simulink model "pathFollowingWithObstacleAvoidanceExample"  (R2020a)
settings: Solver=VariableStepAuto  StartTime=0.0  StopTime=inf  FixedStep=0.01  RelTol=1e-3  EnableMultiTasking=on
undefined symbols (not defined in the file or in its folder): Angular, Linear
libraries: robotlib x4, robotalgslib x2
settings Model: Creator=The MathWorks, Inc.  LastModifiedBy=Param
settings DataIOCC: ReturnWorkspaceOutputs=off
settings DebuggingCC: PregeneratedLibrarySubsystemCodeDiagnostic=none  ArithmeticOperatorsInVariantConditions=warning
settings SFSimCC: SimUseLocalCustomCode=off  CustomCodeUndefinedFunction=UseInterfaceOnly
settings RTWCC: RTWUseLocalCustomCode=off
settings CodeAppCC: StateflowObjectComments=on
settings GRTTargetCC: TargetLangStandard=C89/C90 (ANSI)
settings ConfigComp: CovMetricSettings=dsw  CovHtmlReporting=on  CovSaveCumulativeToWorkspaceVar=on  CovSaveSingleToWorkspaceVar=on  CovExternalEMLEnable=off

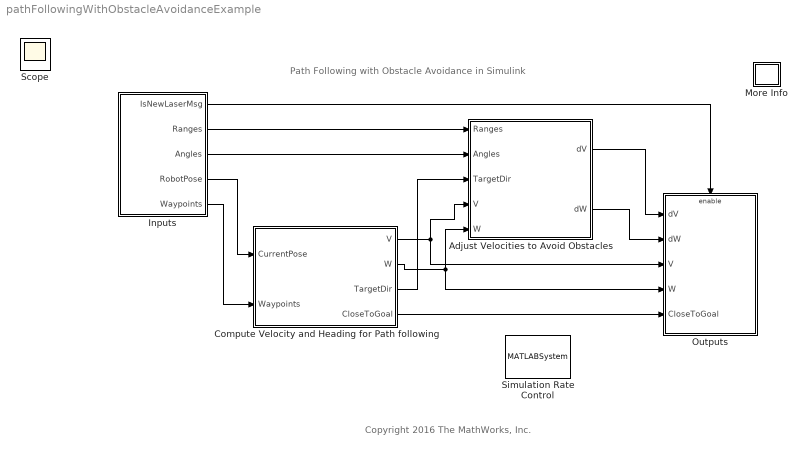
== system pathFollowingWithObstacleAvoidanceExample ==
  note: Path Following with Obstacle Avoidance in Simulink
  note: Copyright 2016 The MathWorks, Inc.
  Adjust Velocities to Avoid Obstacles : Subsystem
  Compute Velocity and Heading for Path following : Subsystem
  Inputs : Subsystem
  More Info : Subsystem
      settings: OpenFcn=showdemo(bdroot(gcb))
      mask Display: disp('?')
  Outputs : Subsystem
  Simulation Rate Control : MATLABSystem  System=ExampleHelperSimulationRateControl  SampleTime=0.02
      mask Type: ExampleHelperSimulationRateControl
      mask Display: disp('Rate Control');
  Scope : Scope
  wires:
  Compute Velocity and Heading for Path following/1(V) -> Outputs/3(V), Adjust Velocities to Avoid Obstacles/4(V)
  Compute Velocity and Heading for Path following/3(TargetDir) -> Adjust Velocities to Avoid Obstacles/3(TargetDir)
  Inputs/2(Ranges) -> Adjust Velocities to Avoid Obstacles/1(Ranges)
  Inputs/3(Angles) -> Adjust Velocities to Avoid Obstacles/2(Angles)
  Inputs/1(IsNewLaserMsg) -> Outputs/Enable
  Inputs/4(RobotPose) -> Compute Velocity and Heading for Path following/1(CurrentPose)
  Inputs/5(Waypoints) -> Compute Velocity and Heading for Path following/2(Waypoints)
  Compute Velocity and Heading for Path following/2(W) -> Outputs/4(W), Adjust Velocities to Avoid Obstacles/5(W)
  Adjust Velocities to Avoid Obstacles/1(dV) -> Outputs/1(dV)
  Adjust Velocities to Avoid Obstacles/2(dW) -> Outputs/2(dW)
  Compute Velocity and Heading for Path following/4(CloseToGoal) -> Outputs/5(CloseToGoal)

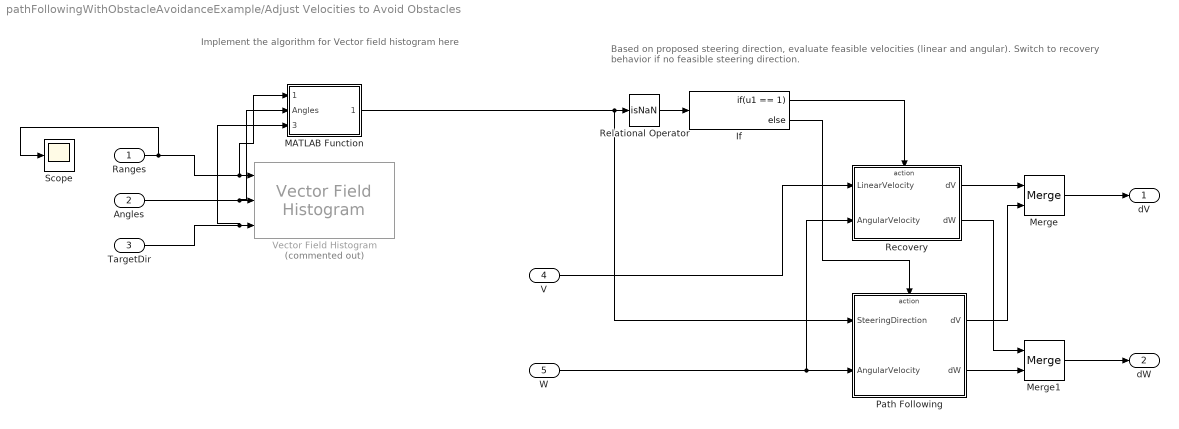
== system pathFollowingWithObstacleAvoidanceExample/Adjust Velocities to Avoid Obstacles ==
  note: Implement the algorithm for Vector field histogram here
  note: Based on proposed steering direction, evaluate feasible velocities (linear and angular).
      | 				Switch to recovery behavior if no feasible steering direction.
  Ranges : Inport
  Angles : Inport  Port=2
  TargetDir : Inport  Port=3
  V : Inport  Port=4
  W : Inport  Port=5
  If : If  IfExpression=u1 == 1
  MATLAB Function : MATLAB Function  TreatAsAtomicUnit=on
  Merge : Merge
  Merge1 : Merge
  Path Following : Subsystem  TreatAsAtomicUnit=on
  Recovery : Subsystem  TreatAsAtomicUnit=on
  Relational Operator : RelationalOperator  Operator=isNaN  OutDataTypeStr=boolean  RndMeth=Simplest
  Scope : Scope
  Vector Field Histogram : robotalgslib/Vector Field Histogram  Commented=on  NumAngularSectors=180  DistanceLimits=[ 0.05, 2 ]  HistogramThresholds=[ 3, 10 ]  RobotRadius=0.1  SafetyDistance=0.1  MinTurningRadius=0.1  SimulateUsing=Code generation  TargetDirectionWeight=5  CurrentDirectionWeight=2  PreviousDirectionWeight=2
      settings: SourceProductBaseCode=NV,RO
  dV : Outport  VectorParamsAs1DForOutWhenUnconnected=off
  dW : Outport  Port=2  VectorParamsAs1DForOutWhenUnconnected=off
  wires:
  Merge1/1 -> dW/1
  V/1 -> Recovery/1(LinearVelocity)
  W/1 -> Recovery/2(AngularVelocity), Path Following/2(AngularVelocity)
  Relational Operator/1 -> If/1
  Merge/1 -> dV/1
  If/1 -> Recovery/Action
  If/2 -> Path Following/Action
  Recovery/2(dW) -> Merge1/1
  Path Following/2(dW) -> Merge1/2
  Recovery/1(dV) -> Merge/1
  Path Following/1(dV) -> Merge/2
  Ranges/1 -> Scope/1, MATLAB Function/1(Ranges), Vector Field Histogram/1
  Angles/1 -> MATLAB Function/2(Angles), Vector Field Histogram/2
  TargetDir/1 -> MATLAB Function/3(TargetDir), Vector Field Histogram/3
  MATLAB Function/1(outangle) -> Path Following/1(SteeringDirection), Relational Operator/1

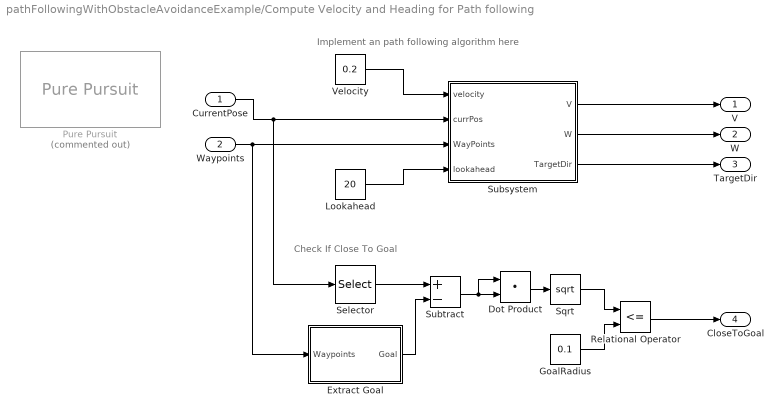
== system pathFollowingWithObstacleAvoidanceExample/Compute Velocity and Heading for Path following ==
  note: Implement an path following algorithm here
  note: Check If Close To Goal
  CurrentPose : Inport
  Waypoints : Inport  Port=2
  " Extract Goal" : MATLAB Function  TreatAsAtomicUnit=on
  Dot Product : DotProduct  InputSameDT=on  OutDataTypeStr=Inherit: Inherit via internal rule
  GoalRadius : Constant  Value=0.1
  Lookahead : Constant  Value=20  OutDataTypeStr=Inherit: Inherit via back propagation
  Pure Pursuit : robotalgslib/Pure Pursuit  Commented=on  DesiredLinearVelocity=0.1  MaxAngularVelocity=1.0  LookaheadDistance=1.0  TargetDirPort=on  SimulateUsing=Code generation
  Relational Operator : RelationalOperator  Operator=<=  OutDataTypeStr=boolean  RndMeth=Simplest
  Selector : Selector  InputPortWidth=3  IndexOptions=Index vector (dialog)  Indices=[1 2]  OutputSizes=1
  Sqrt : Sqrt  SaturateOnIntegerOverflow=on
  Subsystem : Subsystem
  Subtract : Sum  Inputs=+-
  Velocity : Constant  Value=0.2  OutDataTypeStr=Inherit: Inherit via back propagation
  V : Outport  VectorParamsAs1DForOutWhenUnconnected=off
  W : Outport  Port=2  VectorParamsAs1DForOutWhenUnconnected=off
  TargetDir : Outport  Port=3  VectorParamsAs1DForOutWhenUnconnected=off
  CloseToGoal : Outport  Port=4  VectorParamsAs1DForOutWhenUnconnected=off
  wires:
  " Extract Goal"/1(Goal) -> Subtract/2
  Waypoints/1 -> Subsystem/3(WayPoints), " Extract Goal"/1(Waypoints)
  CurrentPose/1 -> Subsystem/2(currPos), Selector/1
  Relational Operator/1 -> CloseToGoal/1
  GoalRadius/1 -> Relational Operator/2
  Selector/1 -> Subtract/1
  Dot Product/1 -> Sqrt/1
  Sqrt/1 -> Relational Operator/1
  Subtract/1 -> Dot Product/1, Dot Product/2
  Velocity/1 -> Subsystem/1(velocity)
  Lookahead/1 -> Subsystem/4(lookahead)
  Subsystem/3(TargetDir) -> TargetDir/1
  Subsystem/1(V) -> V/1
  Subsystem/2(W) -> W/1

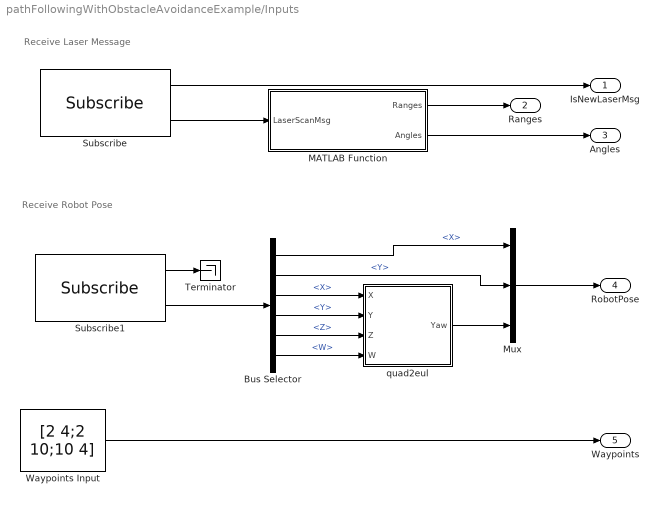
== system pathFollowingWithObstacleAvoidanceExample/Inputs ==
  note: Receive Robot Pose
  note: Receive Laser Message
  Bus Selector : BusSelector  OutputSignals=Pose.Pose.Position.X,Pose.Pose.Position.Y,Pose.Pose.Orientation.X,Pose.Pose.Orientation.Y,Pose.Pose.Orientation.Z,Pose.Pose.Orientation.W
  MATLAB Function : MATLAB Function  TreatAsAtomicUnit=on
  Mux : Mux  Inputs=3
  Subscribe : robotlib/Subscribe  topicSource=Select from ROS network  topic=/scan  messageType=sensor_msgs/LaserScan  sampleTime=-1  messageQueueLength=1
  Subscribe1 : robotlib/Subscribe  topicSource=Select from ROS network  topic=/ground_truth_pose  messageType=nav_msgs/Odometry  sampleTime=-1  messageQueueLength=1
  Terminator : Terminator
  Waypoints Input : Constant  Value=[2 4;2 10;10 4]  VectorParams1D=off  OutDataTypeStr=double
  quad2eul : MATLAB Function  TreatAsAtomicUnit=on
  IsNewLaserMsg : Outport  VectorParamsAs1DForOutWhenUnconnected=off
  Ranges : Outport  Port=2  VectorParamsAs1DForOutWhenUnconnected=off
  Angles : Outport  Port=3  VectorParamsAs1DForOutWhenUnconnected=off
  RobotPose : Outport  Port=4  VectorParamsAs1DForOutWhenUnconnected=off
  Waypoints : Outport  Port=5  VectorParamsAs1DForOutWhenUnconnected=off
  wires:
  Waypoints Input/1 -> Waypoints/1
  Subscribe/2 -> MATLAB Function/1(LaserScanMsg)
  quad2eul/1(Yaw) -> Mux/3
  Subscribe1/2 -> Bus Selector/1
  Bus Selector/3 -> quad2eul/1(X)  "<X>"
  Subscribe1/1 -> Terminator/1
  Bus Selector/2 -> Mux/2  "<Y>"
  Bus Selector/5 -> quad2eul/3(Z)  "<Z>"
  Bus Selector/4 -> quad2eul/2(Y)  "<Y>"
  Bus Selector/1 -> Mux/1  "<X>"
  Bus Selector/6 -> quad2eul/4(W)  "<W>"
  MATLAB Function/1(Ranges) -> Ranges/1
  MATLAB Function/2(Angles) -> Angles/1
  Subscribe/1 -> IsNewLaserMsg/1
  Mux/1 -> RobotPose/1

== system pathFollowingWithObstacleAvoidanceExample/More Info ==

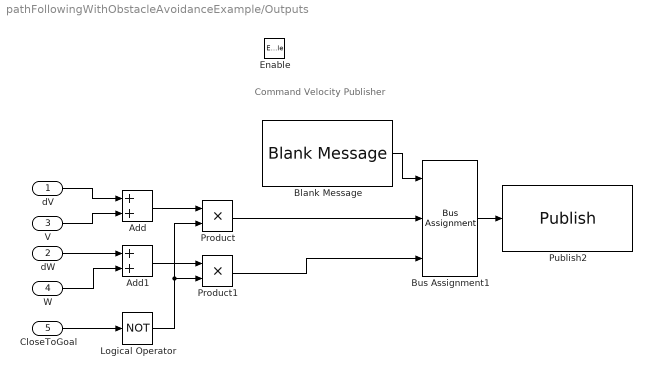
== system pathFollowingWithObstacleAvoidanceExample/Outputs ==
  note: Command Velocity Publisher
  dV : Inport
  dW : Inport  Port=2
  V : Inport  Port=3
  W : Inport  Port=4
  CloseToGoal : Inport  Port=5
  Enable : EnablePort
  Add : Sum
  Add1 : Sum
  Blank Message : robotlib/Blank Message  messageClass=Message  entityType=geometry_msgs/Twist  messageType=geometry_msgs/Twist  SampleTime=inf
  Bus Assignment1 : BusAssignment  DialogController=Simulink.DDGSource_BusAssignment  AssignedSignals=Linear.X,Angular.Z
  Logical Operator : Logic  Operator=NOT  AllPortsSameDT=off  OutDataTypeStr=boolean
  Product : Product
  Product1 : Product
  Publish2 : robotlib/Publish  topicSource=Select from ROS network  topic=/mobile_base/commands/velocity  messageType=geometry_msgs/Twist  messageQueueLength=105
  wires:
  V/1 -> Add/2
  W/1 -> Add1/2
  dV/1 -> Add/1
  dW/1 -> Add1/1
  CloseToGoal/1 -> Logical Operator/1
  Add/1 -> Product/1
  Add1/1 -> Product1/1
  Product1/1 -> Bus Assignment1/3
  Product/1 -> Bus Assignment1/2
  Blank Message/1 -> Bus Assignment1/1
  Bus Assignment1/1 -> Publish2/1
  Logical Operator/1 -> Product1/2, Product/2

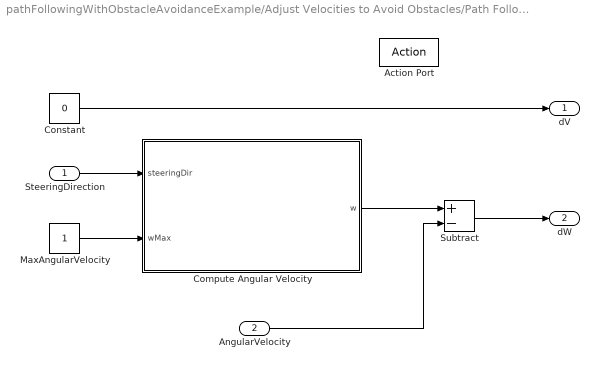
== system pathFollowingWithObstacleAvoidanceExample/Adjust Velocities to Avoid Obstacles/Path Following ==
  SteeringDirection : Inport
  AngularVelocity : Inport  Port=2
  Action Port : ActionPort  ActionPortLabel=else
  Compute Angular Velocity : MATLAB Function  TreatAsAtomicUnit=on
  Constant : Constant  Value=0
  MaxAngularVelocity : Constant
  Subtract : Sum  Inputs=+-
  dV : Outport  VectorParamsAs1DForOutWhenUnconnected=off
  dW : Outport  Port=2  VectorParamsAs1DForOutWhenUnconnected=off
  wires:
  Constant/1 -> dV/1
  MaxAngularVelocity/1 -> Compute Angular Velocity/2(wMax)
  SteeringDirection/1 -> Compute Angular Velocity/1(steeringDir)
  Subtract/1 -> dW/1
  Compute Angular Velocity/1(w) -> Subtract/1
  AngularVelocity/1 -> Subtract/2

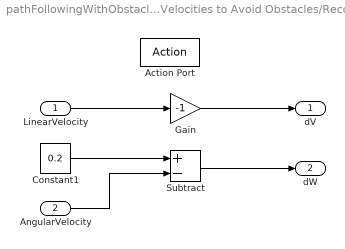
== system pathFollowingWithObstacleAvoidanceExample/Adjust Velocities to Avoid Obstacles/Recovery ==
  LinearVelocity : Inport
  AngularVelocity : Inport  Port=2
  Action Port : ActionPort  ActionPortLabel=if(u1 == 1)
  Constant1 : Constant  Value=0.2
  Gain : Gain  Gain=-1
  Subtract : Sum  Inputs=+-
  dV : Outport  VectorParamsAs1DForOutWhenUnconnected=off
  dW : Outport  Port=2  VectorParamsAs1DForOutWhenUnconnected=off
  wires:
  LinearVelocity/1 -> Gain/1
  Gain/1 -> dV/1
  Constant1/1 -> Subtract/1
  AngularVelocity/1 -> Subtract/2
  Subtract/1 -> dW/1

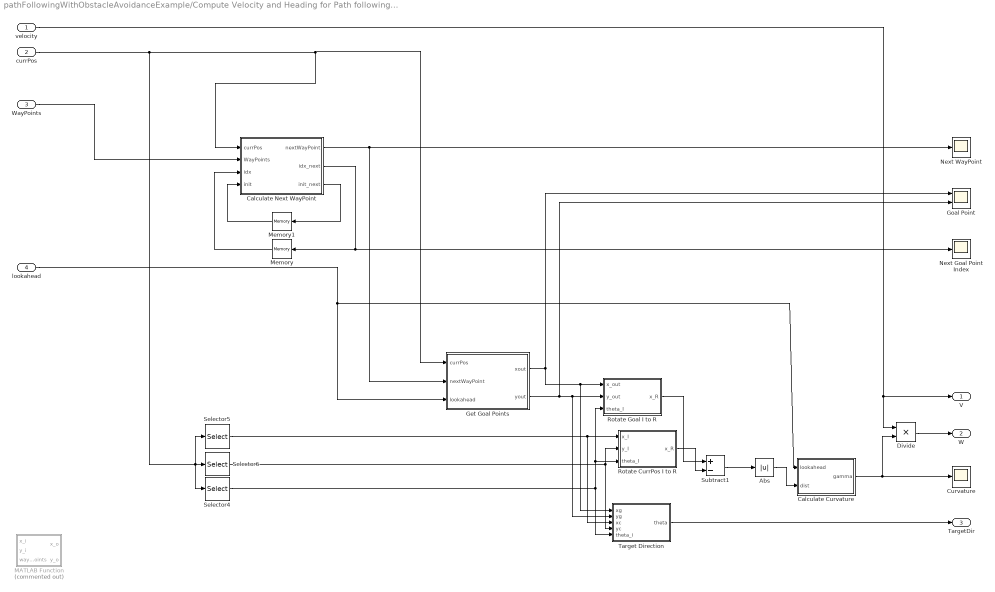
== system pathFollowingWithObstacleAvoidanceExample/Compute Velocity and Heading for Path following/Subsystem ==
  velocity : Inport
  currPos : Inport  Port=2
  WayPoints : Inport  Port=3
  lookahead : Inport  Port=4
  " Rotate CurrPos I to R" : MATLAB Function  TreatAsAtomicUnit=on
  " Rotate Goal I to R" : MATLAB Function  TreatAsAtomicUnit=on
  Abs : Abs
  Calculate Curvature : MATLAB Function  TreatAsAtomicUnit=on
  Calculate Next WayPoint : MATLAB Function  TreatAsAtomicUnit=on
  Curvature : Scope
  Divide : Product  Inputs=**
  Get Goal Points : MATLAB Function  TreatAsAtomicUnit=on
  Goal Point : Scope  NumInputPorts=2
  MATLAB Function : MATLAB Function  Commented=on  TreatAsAtomicUnit=on
  Memory : Memory  InitialCondition=1
  Memory1 : Memory
  Next Goal Point Index : Scope
  Next WayPoint : Scope
  Selector4 : Selector  InputPortWidth=3  IndexOptions=Index vector (dialog)  Indices=[3]  OutputSizes=1
  Selector5 : Selector  InputPortWidth=3  IndexOptions=Index vector (dialog)  Indices=[1]  OutputSizes=1
  Selector6 : Selector  InputPortWidth=3  IndexOptions=Index vector (dialog)  Indices=[2]  OutputSizes=1
  Subtract1 : Sum  Inputs=+-
  Target Direction : MATLAB Function  TreatAsAtomicUnit=on
  V : Outport  VectorParamsAs1DForOutWhenUnconnected=off
  W : Outport  Port=2  VectorParamsAs1DForOutWhenUnconnected=off
  TargetDir : Outport  Port=3  VectorParamsAs1DForOutWhenUnconnected=off
  wires:
  lookahead/1 -> Get Goal Points/3(lookahead), Calculate Curvature/1(lookahead)
  velocity/1 -> V/1, Divide/1
  Calculate Next WayPoint/1(nextWayPoint) -> Get Goal Points/2(nextWayPoint), Next WayPoint/1
  currPos/1 -> Get Goal Points/1(currPos), Calculate Next WayPoint/1(currPos), Selector4/1, Selector5/1, Selector6/1
  Selector5/1 -> " Rotate CurrPos I to R"/1(x_I), Target Direction/3(xc)
  WayPoints/1 -> Calculate Next WayPoint/2(WayPoints)
  Selector4/1 -> Target Direction/5(theta_i), " Rotate CurrPos I to R"/3(theta_I), " Rotate Goal I to R"/3(theta_I)
  Selector6/1 -> " Rotate CurrPos I to R"/2(y_I), Target Direction/4(yc)
  Abs/1 -> Calculate Curvature/2(dist)
  " Rotate Goal I to R"/1(x_R) -> Subtract1/1
  " Rotate CurrPos I to R"/1(x_R) -> Subtract1/2
  Calculate Curvature/1(gamma) -> Divide/2, Curvature/1
  Target Direction/1(theta) -> TargetDir/1
  Subtract1/1 -> Abs/1
  Divide/1 -> W/1
  Calculate Next WayPoint/2(idx_next) -> Next Goal Point Index/1, Memory/1
  Get Goal Points/1(xout) -> " Rotate Goal I to R"/1(x_out), Target Direction/1(xg), Goal Point/1
  Get Goal Points/2(yout) -> " Rotate Goal I to R"/2(y_out), Target Direction/2(yg), Goal Point/2
  Memory/1 -> Calculate Next WayPoint/3(idx)
  Calculate Next WayPoint/3(init_next) -> Memory1/1
  Memory1/1 -> Calculate Next WayPoint/4(init)

== matlab function pathFollowingWithObstacleAvoidanceExample/Compute Velocity and Heading for Path following/Subsystem/Target Direction ==
  data: xg input; yg input; theta output; xc input; yc input; theta_i input
function theta = targetDir(xg,yg,xc,yc,theta_i)
%#codegen
theta = angdiff(theta_i,atan2(yg-yc,xg-xc));
end

== matlab function pathFollowingWithObstacleAvoidanceExample/Adjust Velocities to Avoid Obstacles/MATLAB Function ==
  data: Ranges input; Angles input; TargetDir input; outangle output
function outangle = steeringAngle(Ranges,Angles,TargetDir)
disp("--")
badindices = bitor(isnan(Ranges),isnan(Angles));
Ranges = Ranges(~badindices);
Angles = Angles(~badindices);
a = 15;
b = 1;
Ranges = a-b*Ranges;
numBins = 60; 
edges = linspace(-pi/2,pi/2,numBins+1);
validindices = bitand(Angles >= -pi/2, Angles <= pi/2);
Ranges = Ranges(validindices);
Angles = Angles(validindices);
disp(edges)
[~,edges,bin]=histcounts(Angles,edges);
disp("bin value")
disp(bin)
B = accumarray(bin,Ranges,[numBins 1]);
B = conv(B,1/7*[1 2 3 2 1], 'same');
% B = conv(B,1/11*[1 2 3 4 5 4 3 2 1], 'same');
disp(size(bin))
disp(size(Ranges))
disp("B value")
disp(B)
[~,~,idx]=histcounts(TargetDir,edges);
idx = max(1,idx);
idx = min(idx,numBins);
% minbins with 0 values 
threshold = 15
Bnew = conv(B,1/7*[1 1 1 1 1 1 1], 'same');
disp("Bnew value")
disp(Bnew)
indices = find(Bnew<=threshold);
if isempty(indices)
    outangle = pi/18
else
    [minval, minidx] = min(abs(indices-idx));
        startx = 1;
        endx = size(indices,1);
        if indices(minidx)>=idx
            startx = indices(minidx);
            i = indices(minidx);
            while (Bnew(i)<=threshold & i<size(Bnew))
                endx = i;
                i = i+1;
            end
            outangle = (0.9*edges(startx)+0.1*edges(endx+1))/2;
        else
            endx = indices(minidx);
            i = indices(minidx);
            while (Bnew(i)<=threshold & i>1)
                startx = i;
                i = i-1;
            end
            outangle = (0.1*edges(startx)+0.9*edges(endx+1))/2;
        end
end
disp(idx)
disp(TargetDir)
disp(outangle)

== matlab function pathFollowingWithObstacleAvoidanceExample/Inputs/quad2eul ==
  data: X input; Yaw output; Y input; Z input; W input
function Yaw = quat2eulBlk(X, Y, Z, W)
%#codegen

eularAngles = quat2eul([W, X, Y, Z]);
Yaw = eularAngles(1);

== matlab function pathFollowingWithObstacleAvoidanceExample/Compute Velocity and Heading for Path following/Subsystem/MATLAB Function ==
  data: x_i input; x_o output; y_i input; waypoints input; y_o output
function [x_o, y_o] = pathpoint(x_i, y_i, waypoints)
    distances = pdist2([x_i, y_i],waypoints);
    [minDistance, indexOfMinDistance] = min(distances);
    idx = indexOfMinDistance;
    if indexOfMinDistance == size(waypoints,1)
        idx = idx - 1;
    end
    coefficients = polyfit(distances[indexOfMinDistance],distances[indexOfMinDistance+1], 1);
    m = coefficients(1);
    c = coefficients(2);
    refPath = referencePathFrenet(waypoints);

    
y = u;

== matlab function pathFollowingWithObstacleAvoidanceExample/Compute Velocity and Heading for Path following/Subsystem/ Rotate CurrPos I to R ==
  data: x_I input; y_I input; x_R output; theta_I input
function x_R  = rotation(x_I,y_I,theta_I)
%#codegen
x_R = x_I*cos(theta_I)+y_I*sin(theta_I);
% y_R = -x_I*sin(theta_I)+y_I*cos(theta_I);
% theta_R = theta_I;

== matlab function pathFollowingWithObstacleAvoidanceExample/Compute Velocity and Heading for Path following/Subsystem/Get Goal Points ==
  data: currPos input; xout output; nextWayPoint input; yout output; lookahead input
function [xout,yout] = getGoalPos(currPos,nextWayPoint,lookahead)
x1 = currPos(1);
y1 = currPos(2);
x2 = nextWayPoint(1);
y2 = nextWayPoint(2);
dist = pdist([x1,y1;x2,y2],'euclidean');

if dist<lookahead
    xout = x2;
    yout = y2;
else
    xout = x1+(lookahead/dist)*(x2-x1);
    yout = y1+(lookahead/dist)*(y2-y1);
end
disp("===")
disp([x1,y1;x2,y2;xout,yout])
% eps = 1e-8;
% slope = (y2-y1)/(x2-x1+eps);
% intercpt = (y1*x2-y2*x1)/(x2-x1+eps);

% [xout,yout] = linecirc(slope,intercpt,x1,x2,lookahead);
% fun1 = @(x)(x-x1)^2+(slope*x+intercpt-y1)^2-lookahead^2;
% if fun1(x1)*fun1(x2)>0
%     xout = x2;
%     yout = y2;
% else
%     xout = fzero(fun1,[x1,x2]);
%     yout = slope*xout+intercpt;
% end

== matlab function pathFollowingWithObstacleAvoidanceExample/Inputs/MATLAB Function ==
  data: LaserScanMsg input; Ranges output; Angles output
function [Ranges, Angles] = ExtractRangeData(LaserScanMsg)
%#codegen

% Extract Range information
Ranges = double(LaserScanMsg.Ranges);

% Construct Angles vector using AngleMin and AngleIncrement from sensor
% reading.
angMin = double(LaserScanMsg.AngleMin);
angIncrement = double(LaserScanMsg.AngleIncrement);

numReadings = numel(Ranges);
rawAngles = angMin + (0:numReadings-1)' * angIncrement;

% Wrap the angles to the (-pi,pi] interval.
Angles = robotics.internal.wrapToPi(double(rawAngles));

== matlab function pathFollowingWithObstacleAvoidanceExample/Compute Velocity and Heading for Path following/Subsystem/Calculate Next WayPoint ==
  data: currPos input; nextWayPoint output; WayPoints input; idx input; idx_next output; init input; init_next output
function [nextWayPoint, idx_next, init_next] = nextWayPoint(currPos,WayPoints,idx, init)
init_next = init
if init == 0
    distances = pdist2(currPos(1:2)',WayPoints(idx,:));
    [minDistance, minidx] = min(distances);
    idx = minidx
    init_next = 1
end
idx_next = idx
if norm(currPos(1:2)'-WayPoints(idx,:))<0.1
    idx_next = min(idx + 1, size(WayPoints, 1))
end
nextWayPoint = WayPoints(idx_next,:);
end

== matlab function pathFollowingWithObstacleAvoidanceExample/Compute Velocity and Heading for Path following/ Extract Goal ==
  data: Waypoints input; Goal output
function Goal = extractGoal(Waypoints)
%#codegen
b = isnan(Waypoints);
[rows,~] = find(b);
ridx = setdiff(1:size(Waypoints,1), sort(rows));
Goal = [Waypoints(ridx(end), 1) Waypoints(ridx(end), 2)];

== matlab function pathFollowingWithObstacleAvoidanceExample/Adjust Velocities to Avoid Obstacles/Path Following/Compute Angular Velocity ==
  data: steeringDir input; w output; wMax input
function w = exampleHelperComputeAngularVelocity(steeringDir, wMax)
%EXAMPLEHELPERCOMPUTEANGULARVELOCITY Compute angular velocity
%   W = exampleHelperComputeAngularVelocity(STEERINGDIR)
%   returns the angular velocity W for a differential drive robot in radians
%   per second for a given steering direction STEERINGDIR in the robot's
%   coordinate frame in radians.
%
%   W = exampleHelperComputeAngularVelocity(STEERINGDIR, WMAX)
%   returns the angular velocity W for a differential drive robot in radians
%   per second for a given steering direction STEERINGDIR in the robot's
%   coordinate frame in radians and maximum angular velocity WMAX in
%   radians per second. The output angular velocity is saturated based on
%   the WMAX.
%
%   Example:
%       
%       w = exampleHelperComputeAngularVelocity(0.2, 1);

% Copyright 2015 The MathWorks, Inc.

%#codegen
%#ok<*EMCA>

% Allow variable input arguments
if nargin == 1   
    wMax = inf;
end

validateattributes(steeringDir, {'double'},{'real'},...
    'exampleHelperComputeAngularVelocity', 'STEERINGDIR', 1);
validateattributes(wMax, {'double'},{'real', 'positive'},...
    'exampleHelperComputeAngularVelocity', 'WMAX', 2);

% Computing in robot's coordinate frame
curPose = [0 0 0];

% The following computation is similar to robotics.PurePursuit
lookaheadPoint = [cos(steeringDir), sin(steeringDir)];
slope = atan2((lookaheadPoint(2) - curPose(2)), ...
    (lookaheadPoint(1) - curPose(1)));
alpha = angdiff(curPose(3), slope);

% Angular velocity command for a differential drive robot is
% equal to the desired curvature to be followed by the robot.

w = (2*sin(alpha));

% Pick a constant rotation when robot is facing in the opposite
% direction of the path
if abs(abs(alpha) - pi) < 1e-12
    w = sign(w)*1;
end

if abs(w) > wMax
    w = sign(w)*wMax;
end

end

== matlab function pathFollowingWithObstacleAvoidanceExample/Compute Velocity and Heading for Path following/Subsystem/ Rotate Goal I to R ==
  data: x_out input; y_out input; x_R output; theta_I input
function x_R  = rotation(x_out,y_out,theta_I)
%#codegen
x_R = x_out*cos(theta_I)+y_out*sin(theta_I);
% y_R = -x_out*sin(theta_I)+y_out*cos(theta_I);
% theta_R = theta_I;

== matlab function pathFollowingWithObstacleAvoidanceExample/Compute Velocity and Heading for Path following/Subsystem/Calculate Curvature ==
  data: lookahead input; dist input; gamma output
function gamma = curvature(lookahead,dist)
%#codegen
gamma = 2*dist/(lookahead^2);
